simulink library "lib_GenTools_3DlinearInterp"  (R2015a)
settings: Solver=ode45  StartTime=0.0  StopTime=10.0  RelTol=1e-3
settings Model: Creator=jlkratz  LastModifiedBy=jlkratz

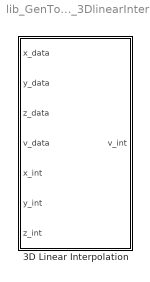
== system lib_GenTools_3DlinearInterp ==
  3D Linear Interpolation : Subsystem  mask(TSAT - 3D Linear Interpolation Block){BN_M=double(gcb)}
      mask prompts: BN_M "BN_M - Block Name"
      mask help: This block performs linear interpolation on a set of data v_data = f(y_data,x_data,z_data) at interpolation points defined in the arrays x_int, y_int, and z_int.
      mask Help: web(which('GenTools_TSAT_3DlinearInterp.html'),'-helpbrowser')

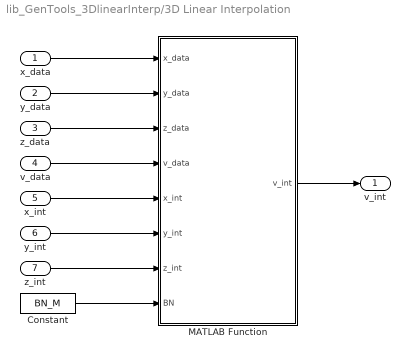
== system lib_GenTools_3DlinearInterp/3D Linear Interpolation ==
  x_data : Inport
  y_data : Inport  Port=2
  z_data : Inport  Port=3
  v_data : Inport  Port=4
  x_int : Inport  Port=5
  y_int : Inport  Port=6
  z_int : Inport  Port=7
  Constant : Constant  Value=BN_M
  MATLAB Function : MATLAB Function  TreatAsAtomicUnit=on
  v_int : Outport
  wires:
  z_int/1 -> MATLAB Function/7(z_int)
  v_data/1 -> MATLAB Function/4(v_data)
  y_int/1 -> MATLAB Function/6(y_int)
  z_data/1 -> MATLAB Function/3(z_data)
  x_int/1 -> MATLAB Function/5(x_int)
  MATLAB Function/1(v_int) -> v_int/1
  y_data/1 -> MATLAB Function/2(y_data)
  Constant/1 -> MATLAB Function/8(BN)
  x_data/1 -> MATLAB Function/1(x_data)

== matlab function lib_GenTools_3DlinearInterp/3D Linear Interpolation/MATLAB Function ==
  data: x_data input; y_data input; z_data input; v_data input; x_int input; y_int input; z_int input; BN input; v_int output
function v_int = interp3D(x_data,y_data,z_data,v_data,x_int,y_int,z_int,BN)
%#codegen

[n1,m1] = size(x_data);
[n2,m2] = size(y_data);
[n3,m3] = size(z_data);
[n4,m4,o4] = size(v_data);
[n5,m5] = size(x_int);
[n6,m6] = size(y_int);
[n7,m7] = size(z_int);
diff_xdata = diff(x_data);
diff_ydata = diff(y_data);
diff_zdata = diff(z_data);

if min([n1,m1]) ~= 1
    v_int = ones(n5,m5);
    fprintf('Warning in %s: x_data must be a 1-D array. v_int has been set to an array of ones the size of x_int as a default.\n',char(BN));
elseif min([n2,m2]) ~= 1
    v_int = ones(n5,m5);
    fprintf('Warning in %s: y_data must be a 1-D array. v_int has been set to an array of ones the size of x_int as a default.\n',char(BN));
elseif min([n3,m3]) ~= 1
    v_int = ones(n5,m5);
    fprintf('Warning in %s: z_data must be a 1-D array. v_int has been set to an array of ones the size of x_int as a default.\n',char(BN));
elseif n4 ~= max([n2,m2]) || m4 ~= max([n1,m1]) || o4 ~= max([n3,m3])
    v_int = ones(n5,m5);
    fprintf('Warning in %s: v_data must be a 3-D array with as many rows as elements in y_data, as many columns as elements in x_data, and as many levels at elements in z_data. v_int has been set to an array of ones the size of x_int as a default.\n',char(BN));
elseif min([n5,m5]) ~= 1
    v_int = ones(n5,m5);
    fprintf('Warning in %s: x_int must be a 1-D array. v_int has been set to an array of ones the size of x_int as a default.\n',char(BN));
elseif min([n6,m6]) ~= 1
    v_int = ones(n5,m5);
    fprintf('Warning in %s: y_int must be a 1-D array. v_int has been set to an array of ones the size of x_int as a default.\n',char(BN));
elseif min([n7,m7]) ~= 1
    v_int = ones(n5,m5);
    fprintf('Warning in %s: z_int must be a 1-D array. v_int has been set to an array of ones the size of x_int as a default.\n',char(BN));
elseif (n5 ~= n6) || (m5 ~= m6) || (n5 ~= n7) || (m5 ~= m7)
    v_int = ones(n5,m5);
    fprintf('Warning in %s: x_int, y_int, and z_int must have the same dimensions. v_int has been set to an array of ones the size of x_int as a default.\n',char(BN));
elseif min(diff_xdata) <= 0
    v_int = ones(n5,m5);
    fprintf('Warning in %s: x_data must be monotonically increasing. v_int has been set to an array of ones the size of x_int as a default.\n',char(BN));
elseif min(diff_ydata) <= 0
    v_int = ones(n5,m5);
    fprintf('Warning in %s: y_data must be monotonically increasing. v_int has been set to an array of ones the size of x_int as a default.\n',char(BN));
elseif min(diff_zdata) <= 0
    v_int = ones(n5,m5);
    fprintf('Warning in %s: y_data must be monotonically increasing. v_int has been set to an array of ones the size of x_int as a default.\n',char(BN));
else
    v_int = zeros(n5,m5);
    for i = 1:length(x_int)
        if x_int(i) < x_data(1)
            if y_int(i) < y_data(1)
                %x_int < x_data(1)   && y_int < y_data(1)   && z_int < z_data(1)
                if z_int(i) < z_data(1)
                    v_int(i) = v_data(1,1,1);
                    fprintf('Warning in %s: x_int(%-1.0i) < x_data(1), y_int(%-1.0i) < y_data(1), and z_int(%-1.0i) < z_data(1). v_int(%-1.0i) has been set to the value of the closest data point.\n',char(BN),int8(i),int8(i),int8(i),int8(i));
                %x_int < x_data(1)   && y_int < y_data(1)   && z_int > z_data(end)
                elseif z_int(i) > z_data(end)
                    v_int(i) = v_data(1,1,end);
                    fprintf('Warning in %s: x_int(%-1.0i) < x_data(1), y_int(%-1.0i) < y_data(1), and z_int(%-1.0i) > z_data(end). v_int(%-1.0i) has been set to the value of the closest data point.\n',char(BN),int8(i),int8(i),int8(i),int8(i));
                %x_int < x_data(1)   && y_int < y_data(1)   && z_int is in range
                else
                    v_temp = zeros(1,length(z_data));
                    for j = 1:length(v_temp)
                        v_temp(j) = v_data(1,1,j);
                    end
                    v_int(i) = interp1(z_data,v_temp,z_int(i));
                    fprintf('Warning in %s: x_int(%-1.0i) < x_data(1) and y_int(%-1.0i) < y_data(1). v_int(%-1.0i) has been interpolated from data on the closest edge of the defined domain.\n',char(BN),int8(i),int8(i),int8(i));
                end
            elseif y_int(i) > y_data(end)
                %x_int < x_data(1)   && y_int > y_data(end) && z_int < z_data(1)
                if z_int(i) < z_data(1)
                    v_int(i) = v_data(end,1,1);
                    fprintf('Warning in %s: x_int(%-1.0i) < x_data(1), y_int(%-1.0i) > y_data(end), and z_int(%-1.0i) < z_data(1). v_int(%-1.0i) has been set to the value of the closest data point.\n',char(BN),int8(i),int8(i),int8(i),int8(i));
                %x_int < x_data(1)   && y_int > y_data(end) && z_int > z_data(end)
                elseif z_int(i) > z_data(end)
                    v_int(i) = v_data(end,1,end);
                    fprintf('Warning in %s: x_int(%-1.0i) < x_data(1), y_int(%-1.0i) > y_data(end), and z_int(%-1.0i) > z_data(end). v_int(%-1.0i) has been set to the value of the closest data point.\n',char(BN),int8(i),int8(i),int8(i),int8(i));
                %x_int < x_data(1)   && y_int > y_data(end) && z_int is in range
                else
                    v_temp = zeros(1,length(z_data));
                    for j = 1:length(v_temp)
                        v_temp(j) = v_data(end,1,j);
                    end
                    v_int(i) = interp1(z_data,v_temp,z_int(i));
                    fprintf('Warning in %s: x_int(%-1.0i) < x_data(1) and y_int(%-1.0i) > y_data(end). v_int(%-1.0i) has been interpolated from data on the closest edge of the defined domain.\n',char(BN),int8(i),int8(i),int8(i));
                end
            else
                %x_int < x_data(1)   && y_int is in range   && z_int < z_data(1)
                if z_int(i) < z_data(1)
                    v_temp = zeros(1,length(y_data));
                    for j = 1:length(v_temp)
                        v_temp(j) = v_data(j,1,1);
                    end
                    v_int(i) = interp1(y_data,v_temp,y_int(i));
                    fprintf('Warning in %s: x_int(%-1.0i) < x_data(1) and z_int(%-1.0i) < z_data(1). v_int(%-1.0i) has been interpolated from data on the closest edge of the defined domain.\n',char(BN),int8(i),int8(i),int8(i));
                %x_int < x_data(1)   && y_int is in range   && z_int > z_data(end)
                elseif z_int(i) > z_data(end)
                    v_temp = zeros(1,length(y_data));
                    for j = 1:length(v_temp)
                        v_temp(j) = v_data(j,1,end);
                    end
                    v_int(i) = interp1(y_data,v_temp,y_int(i));
                    fprintf('Warning in %s: x_int(%-1.0i) < x_data(1) and z_int(%-1.0i) > z_data(end). v_int(%-1.0i) has been interpolated from data on the closest edge of the defined domain.\n',char(BN),int8(i),int8(i),int8(i));
                %x_int < x_data(1)   && y_int is in range   && z_int is in range
                else
                    v_temp = zeros(length(z_data),length(y_data));
                    for j = 1:length(z_data)
                        for k = 1:length(y_data)
                            v_temp(j,k) = v_data(k,1,j);
                        end
                    end
                    v_int(i) = interp2(y_data,z_data,v_temp,y_int(i),z_int(i));
                    fprintf('Warning in %s: x_int(%-1.0i) < x_data(1). v_int(%-1.0i) has been interpolated from data on the closest surface of the defined domain.\n',char(BN),int8(i),int8(i));
                end
            end
        elseif x_int(i) > x_data(end)
            if y_int(i) < y_data(1)
                %x_int > x_data(end) && y_int < y_data(1)   && z_int < z_data(1)
                if z_int(i) < z_data(1)
                    v_int(i) = v_data(1,end,1);
                    fprintf('Warning in %s: x_int(%-1.0i) > x_data(end), y_int(%-1.0i) < y_data(1), and z_int(%-1.0i) < z_data(1). v_int(%-1.0i) has been set to the value of the closest data point.\n',char(BN),int8(i),int8(i),int8(i),int8(i));
                %x_int > x_data(end) && y_int < y_data(1)   && z_int > z_data(end)
                elseif z_int(i) > z_data(end)
                    v_int(i) = v_data(1,end,end);
                    fprintf('Warning in %s: x_int(%-1.0i) > x_data(end), y_int(%-1.0i) < y_data(1), and z_int(%-1.0i) > z_data(end). v_int(%-1.0i) has been set to the value of the closest data point.\n',char(BN),int8(i),int8(i),int8(i),int8(i));
                %x_int > x_data(end) && y_int < y_data(1)   && z_int is in range
                else
                    v_temp = zeros(1,length(z_data));
                    for j = 1:length(v_temp)
                        v_temp(j) = v_data(1,end,j);
                    end
                    v_int(i) = interp1(z_data,v_temp,z_int(i));
                    fprintf('Warning in %s: x_int(%-1.0i) > x_data(end) and y_int(%-1.0i) < y_data(1). v_int(%-1.0i) has been interpolated from data on the closest edge of the defined domain.\n',char(BN),int8(i),int8(i),int8(i));
                end
            elseif y_int(i) > y_data(end)
                %x_int > x_data(end) && y_int > y_data(end) && z_int < z_data(1)
                if z_int(i) < z_data(1)
                    v_int(i) = v_data(end,end,1);
                    fprintf('Warning in %s: x_int(%-1.0i) > x_data(end), y_int(%-1.0i) > y_data(end), and z_int(%-1.0i) < z_data(1). v_int(%-1.0i) has been set to the value of the closest data point.\n',char(BN),int8(i),int8(i),int8(i),int8(i));
                %x_int > x_data(end) && y_int > y_data(end) && z_int > z_data(end)
                elseif z_int(i) > z_data(end)
                    v_int(i) = v_data(end,end,end);
                    fprintf('Warning in %s: x_int(%-1.0i) > x_data(end), y_int(%-1.0i) > y_data(end), and z_int(%-1.0i) > z_data(end). v_int(%-1.0i) has been set to the value of the closest data point.\n',char(BN),int8(i),int8(i),int8(i),int8(i));
                %x_int > x_data(end) && y_int > y_data(end) && z_int is in range
                else
                    v_temp = zeros(1,length(z_data));
                    for j = 1:length(v_temp)
                        v_temp(j) = v_data(end,end,j);
                    end
                    v_int(i) = interp1(z_data,v_temp,z_int(i));
                    fprintf('Warning in %s: x_int(%-1.0i) > x_data(end) and y_int(%-1.0i) > y_data(end). v_int(%-1.0i) has been interpolated from data on the closest edge of the defined domain.\n',char(BN),int8(i),int8(i),int8(i));
                end
            else
                %x_int > x_data(end) && y_int is in range   && z_int < z_data(1)
                if z_int(i) < z_data(1)
                    v_temp = zeros(1,length(y_data));
                    for j = 1:length(v_temp)
                        v_temp(j) = v_data(j,end,1);
                    end
                    v_int(i) = interp1(y_data,v_temp,y_int(i));
                    fprintf('Warning in %s: x_int(%-1.0i) > x_data(end) and z_int(%-1.0i) < z_data(1). v_int(%-1.0i) has been interpolated from data on the closest edge of the defined domain.\n',char(BN),int8(i),int8(i),int8(i));
                %x_int > x_data(end) && y_int is in range   && z_int > z_data(end)
                elseif z_int(i) > z_data(end)
                    v_temp = zeros(1,length(y_data));
                    for j = 1:length(v_temp)
                        v_temp(j) = v_data(j,end,end);
                    end
                    v_int(i) = interp1(y_data,v_temp,y_int(i));
                    fprintf('Warning in %s: x_int(%-1.0i) > x_data(end) and z_int(%-1.0i) > z_data(end). v_int(%-1.0i) has been interpolated from data on the closest edge of the defined domain.\n',char(BN),int8(i),int8(i),int8(i));
                %x_int > x_data(end) && y_int is in range   && z_int is in range
                else
                    v_temp = zeros(length(z_data),length(y_data));
                    for j = 1:length(z_data)
                        for k = 1:length(y_data)
                            v_temp(j,k) = v_data(k,end,j);
                        end
                    end
                    v_int(i) = interp2(y_data,z_data,v_temp,y_int(i),z_int(i));
                    fprintf('Warning in %s: x_int(%-1.0i) > x_data(end). v_int(%-1.0i) has been interpolated from data on the closest surface of the defined domain.\n',char(BN),int8(i),int8(i));
                end
            end
        else
            if y_int(i) < y_data(1)
                %x_int is in range   && y_int < y_data(1)   && z_int < z_data(1)
                if z_int(i) < z_data(1)
                    v_temp = zeros(1,length(x_data));
                    for j = 1:length(v_temp)
                        v_temp(j) = v_data(1,j,1);
                    end
                    v_int(i) = interp1(x_data,v_temp,x_int(i));
                    fprintf('Warning in %s: y_int(%-1.0i) < y_data(1) and z_int(%-1.0i) < z_data(1). v_int(%-1.0i) has been interpolated from data on the closest edge of the defined domain.\n',char(BN),int8(i),int8(i),int8(i));
                %x_int is in range   && y_int < y_data(1)   && z_int > z_data(end)
                elseif z_int(i) > z_data(end)
                    v_temp = zeros(1,length(x_data));
                    for j = 1:length(v_temp)
                        v_temp(j) = v_data(1,j,end);
                    end
                    v_int(i) = interp1(x_data,v_temp,x_int(i));
                    fprintf('Warning in %s: y_int(%-1.0i) < y_data(1) and z_int(%-1.0i) > z_data(end). v_int(%-1.0i) has been interpolated from data on the closest edge of the defined domain.\n',char(BN),int8(i),int8(i),int8(i));
                %x_int is in range   && y_int < y_data(1)   && z_int is in range
                else
                    v_temp = zeros(length(z_data),length(x_data));
                    for j = 1:length(z_data)
                        for k = 1:length(x_data)
                            v_temp(j,k) = v_data(1,k,j);
                        end
                    end
                    v_int(i) = interp2(x_data,z_data,v_temp,x_int(i),z_int(i));
                    fprintf('Warning in %s: y_int(%-1.0i) < y_data(1). v_int(%-1.0i) has been interpolated from data on the closest surface of the defined domain.\n',char(BN),int8(i),int8(i));
                end
            elseif y_int(i) > y_data(end)
                %x_int is in range   && y_int > y_data(end) && z_int < z_data(1)
                if z_int(i) < z_data(1)
                    v_temp = zeros(1,length(x_data));
                    for j = 1:length(v_temp)
                        v_temp(j) = v_data(end,j,1);
                    end
                    v_int(i) = interp1(x_data,v_temp,x_int(i));
                    fprintf('Warning in %s: y_int(%-1.0i) > y_data(end) and z_int(%-1.0i) < z_data(1). v_int(%-1.0i) has been interpolated from data on the closest edge of the defined domain.\n',char(BN),int8(i),int8(i),int8(i));
                %x_int is in range   && y_int > y_data(end) && z_int > z_data(end)
                elseif z_int(i) > z_data(end)
                    v_temp = zeros(1,length(x_data));
                    for j = 1:length(v_temp)
                        v_temp(j) = v_data(end,j,end);
                    end
                    v_int(i) = interp1(x_data,v_temp,x_int(i));
                    fprintf('Warning in %s: y_int(%-1.0i) > y_data(end) and z_int(%-1.0i) > z_data(end). v_int(%-1.0i) has been interpolated from data on the closest edge of the defined domain.\n',char(BN),int8(i),int8(i),int8(i));
                %x_int is in range   && y_int > y_data(end) && z_int is in range
                else
                    v_temp = zeros(length(z_data),length(x_data));
                    for j = 1:length(z_data)
                        for k = 1:length(x_data)
                            v_temp(j,k) = v_data(end,k,j);
                        end
                    end
                    v_int(i) = interp2(x_data,z_data,v_temp,x_int(i),z_int(i));
                    fprintf('Warning in %s: y_int(%-1.0i) > y_data(end). v_int(%-1.0i) has been interpolated from data on the closest surface of the defined domain.\n',char(BN),int8(i),int8(i));
                end
            else
                %x_int is in range   && y_int is in range   && z_int < z_data(1)
                if z_int(i) < z_data(1)
                    v_temp = zeros(length(y_data),length(x_data));
                    for j = 1:length(y_data)
                        for k = 1:length(x_data)
                            v_temp(j,k) = v_data(j,k,1);
                        end
                    end
                    v_int(i) = interp2(x_data,y_data,v_temp,x_int(i),y_int(i));
                    fprintf('Warning in %s: z_int(%-1.0i) < z_data(1). v_int(%-1.0i) has been interpolated from data on the closest surface of the defined domain.\n',char(BN),int8(i),int8(i));
                %x_int is in range   && y_int is in range   && z_int > z_data(end)
                elseif z_int(i) > z_data(end)
                    v_temp = zeros(length(y_data),length(x_data));
                    for j = 1:length(y_data)
                        for k = 1:length(x_data)
                            v_temp(j,k) = v_data(j,k,end);
                        end
                    end
                    v_int(i) = interp2(x_data,y_data,v_temp,x_int(i),y_int(i));
                    fprintf('Warning in %s: z_int(%-1.0i) > z_data(end). v_int(%-1.0i) has been interpolated from data on the closest surface of the defined domain.\n',char(BN),int8(i),int8(i));
                %x_int is in range   && y_int is in range   && z_int is in range
                else
                    v_int(i) = interp3(x_data,y_data,z_data,v_data,x_int(i),y_int(i),z_int(i));
                end
            end
        end
    end
end
